simulink model "Exercitii_Laborator"  (R2016a)
settings: Solver=VariableStepDiscrete  StartTime=0.0  StopTime=40  RelTol=1e-3
undefined symbols (not defined in the file): m, n
settings Model: Creator=Cristina  LastModifiedBy=Cristina

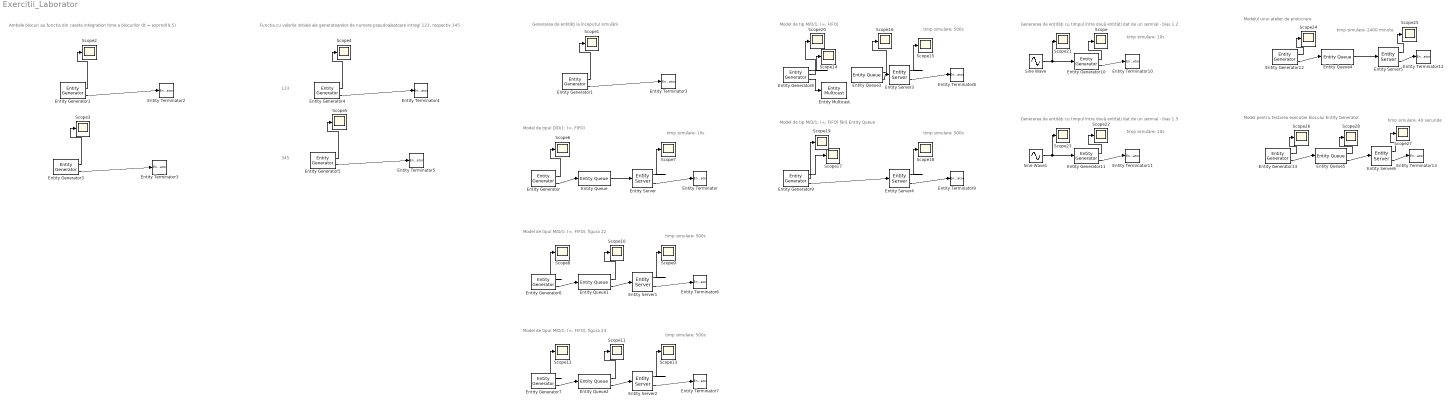
== system Exercitii_Laborator ==
  note: Model pentru testarea execuției blocului Entity Generator
  note: Generarea de entități cu timpul între două entități dat de un semnal - bias 1.2
  note: timp simulare: 10s
  note: Model de tipul D/D/1: (∞, FIFO)
  note: Generarea de entități la începutul simulării
  note: 345
  note: 123
  note: Functia cu valorile initiale ale generatoarelor de numere pseudoaleatoare intregi 123, respectiv
      | 345
  note: Ambele blocuri au functia din caseta integration time a blocurilor dt = exprnd(0.5)
  note: Model de tipul M/D/1: (∞, FIFO), figura 22
  note: timp simulare: 500s
  note: Model de tipul M/D/1: (∞, FIFO), figura 23
  note: timp simulare: 500s
  note: timp simulare: 500s
  note: Model de tip M/D/1; (∞, FIFO)
  note: timp simulare: 500s
  note: Model de tip M/D/1; (∞, FIFO) fără Entity Queue
  note: timp simulare: 10s
  note: Generarea de entități cu timpul între două entități dat de un semnal - bias 1.5
  note: timp simulare: 10s
  note: Modelul unui atelier de prelucrare
  note: timp simulare: 2400 minute
  note: timp simulare: 40 secunde
  Entity Generator : EntityGenerator  OutputPortMessageModes=n,m  NumberEntitiesDeparted=on  EntityType=Structured  EntityTypeName=Entity
      settings: OutputPortMap=o0,o3
  Entity Generator1 : EntityGenerator  OutputPortMessageModes=n,m  TimeSource=MATLAB action  IntergenerationTimeAction=|  NumberEntitiesDeparted=on  EntityType=Structured  EntityTypeName=Entity
      | persistent count
      | if (isempty(count))
      |     count = 1;
      | end
      | 
      | if count < 10
      |     dt = 0;
      |     count = count + 1;
      | else
      |     dt = inf;
      | end
      settings: OutputPortMap=o0,o3
  Entity Generator10 : EntityGenerator  OutputPortMessageModes=n,m  TimeSource=Signal port  NumberEntitiesDeparted=on  EntityType=Structured  EntityTypeName=Entity
      settings: InputPortMap=u1  OutputPortMap=o0,o3
  Entity Generator11 : EntityGenerator  OutputPortMessageModes=n,m  TimeSource=Signal port  NumberEntitiesDeparted=on  EntityType=Structured  EntityTypeName=Entity
      settings: InputPortMap=u1  OutputPortMap=o0,o3
  Entity Generator12 : EntityGenerator  OutputPortMessageModes=n,m  TimeSource=MATLAB action  IntergenerationTimeAction=|  AverageIntergenerationTime=on  EntityType=Structured  EntityTypeName=Entity
      | persistent init
      | if (isempty(init))
      |     rng(1957);
      |     init = true;
      | end
      | dt = 1 + rand * 12;
      settings: OutputPortMap=o2,o3
  Entity Generator13 : EntityGenerator  OutputPortMessageModes=n,m  IntergenerationTimeAction=|  NumberEntitiesDeparted=on  EntityType=Structured  EntityTypeName=Entity
      | persistent init
      | if (isempty(init))
      |     rng(1957);
      |     init = true;
      | end
      | dt = 1 + rand * 12;
      settings: OutputPortMap=o0,o3
  Entity Generator2 : EntityGenerator  OutputPortMessageModes=n,m  TimeSource=MATLAB action  IntergenerationTimeAction=dt = exprnd(0.5);  NumberEntitiesDeparted=on  EntityType=Structured  EntityTypeName=Entity
      settings: OutputPortMap=o0,o3
  Entity Generator3 : EntityGenerator  OutputPortMessageModes=n,m  TimeSource=MATLAB action  IntergenerationTimeAction=dt = exprnd(0.5);  NumberEntitiesDeparted=on  EntityType=Structured  EntityTypeName=Entity
      settings: OutputPortMap=o0,o3
  Entity Generator4 : EntityGenerator  OutputPortMessageModes=n,m  TimeSource=MATLAB action  IntergenerationTimeAction=|  NumberEntitiesDeparted=on  EntityType=Structured  EntityTypeName=Entity
      | persistent init
      | if isempty(init)
      |     rng(123);
      |     init = true;
      | end
      | 
      | dt = exprnd(0.5);
      settings: OutputPortMap=o0,o3
  Entity Generator5 : EntityGenerator  OutputPortMessageModes=n,m  TimeSource=MATLAB action  IntergenerationTimeAction=|  NumberEntitiesDeparted=on  EntityType=Structured  EntityTypeName=Entity
      | persistent init
      | if isempty(init)
      |     rng(345);
      |     init = true;
      | end
      | 
      | dt = exprnd(0.5);
      settings: OutputPortMap=o0,o3
  Entity Generator6 : EntityGenerator  OutputPortMessageModes=n,m  TimeSource=MATLAB action  IntergenerationTimeAction=dt = exprnd(0.5);  AverageIntergenerationTime=on  EntityType=Structured  EntityTypeName=Entity
      settings: OutputPortMap=o2,o3
  Entity Generator7 : EntityGenerator  OutputPortMessageModes=n,m  TimeSource=MATLAB action  IntergenerationTimeAction=|  AverageIntergenerationTime=on  EntityType=Structured  EntityTypeName=Entity
      | persistent init
      | if (isempty(init))
      |     rng(1437);
      |     init = true;
      | end
      | dt = exprnd(0.5);
      settings: OutputPortMap=o2,o3
  Entity Generator8 : EntityGenerator  OutputPortMessageModes=n,n,m  TimeSource=MATLAB action  IntergenerationTimeAction=|  NumberEntitiesDeparted=on  AverageIntergenerationTime=on  EntityType=Structured  EntityTypeName=Entity
      | persistent init
      | if (isempty(init))
      |     rng(1437);
      |     init = true;
      | end
      | dt = exprnd(0.5);
      settings: OutputPortMap=o0,o2,o3
  Entity Generator9 : EntityGenerator  OutputPortMessageModes=n,n,m  TimeSource=MATLAB action  IntergenerationTimeAction=|  NumberEntitiesDeparted=on  AverageIntergenerationTime=on  EntityType=Structured  EntityTypeName=Entity
      | persistent init
      | if (isempty(init))
      |     rng(1437);
      |     init = true;
      | end
      | dt = exprnd(0.5);
      settings: OutputPortMap=o0,o2,o3
  Entity Multicast : EntityMulticast  InputPortMessageModes=m
  Entity Queue : EntityQueue  InputPortMessageModes=m  OutputPortMessageModes=m
      settings: OutputPortMap=o5
  Entity Queue1 : EntityQueue  InputPortMessageModes=m  OutputPortMessageModes=n,m  NumberEntitiesInBlock=on
      settings: OutputPortMap=o1,o5
  Entity Queue2 : EntityQueue  InputPortMessageModes=m  OutputPortMessageModes=n,m  NumberEntitiesInBlock=on
      settings: OutputPortMap=o1,o5
  Entity Queue3 : EntityQueue  OutputPortMessageModes=n,m  EntityArrivalSource=Multicast  NumberEntitiesInBlock=on
      settings: OutputPortMap=o1,o5
  Entity Queue4 : EntityQueue  InputPortMessageModes=m  OutputPortMessageModes=m
      settings: OutputPortMap=o5
  Entity Queue5 : EntityQueue  InputPortMessageModes=m  OutputPortMessageModes=n,m  Capacity=10  NumberEntitiesInBlock=on
      settings: OutputPortMap=o1,o5
  Entity Server : EntityServer  InputPortMessageModes=m  OutputPortMessageModes=n,m  Capacity=1  NumberEntitiesDeparted=on
      settings: OutputPortMap=o0,o9
  Entity Server{1..4} (4 alike) : EntityServer  InputPortMessageModes=m  OutputPortMessageModes=n,m  Capacity=1  ServiceTimeValue=0.5  AverageWait=on
      settings: OutputPortMap=o4,o9
  Entity Server5 : EntityServer  InputPortMessageModes=m  OutputPortMessageModes=n,m  Capacity=1  ServiceTimeSource=MATLAB action  ServiceTimeAction=|  AverageWait=on
      | persistent init
      | if (isempty(init))
      |     rng(2347);
      |     init = true;
      | end
      | dt = 3.5 + rand * 3;
      settings: OutputPortMap=o4,o9
  Entity Server6 : EntityServer  InputPortMessageModes=m  OutputPortMessageModes=n,m  Capacity=1  ServiceTimeValue=2  ServiceTimeAction=|  NumberEntitiesDeparted=on
      | persistent init
      | if (isempty(init))
      |     rng(2347);
      |     init = true;
      | end
      | dt = 3.5 + rand * 3;
      settings: OutputPortMap=o0,o9
  Entity Terminator{,1..13} (14 alike) : EntityTerminator  InputPortMessageModes=m
  Scope{,1..28} (29 alike) : Scope
  Sine Wave : Sin  Bias=1.2  Frequency=1.2  SampleTime=0
  Sine Wave1 : Sin  Bias=1.5  Frequency=1.2  SampleTime=0
  wires:
  Entity Generator2/2 -> Entity Terminator2/1
  Entity Generator2/1 -> Scope2/1
  Entity Generator3/2 -> Entity Terminator3/1
  Entity Generator3/1 -> Scope3/1
  Entity Generator4/2 -> Entity Terminator4/1
  Entity Generator4/1 -> Scope4/1
  Entity Generator5/2 -> Entity Terminator5/1
  Entity Generator5/1 -> Scope5/1
  Entity Generator1/2 -> Entity Terminator1/1
  Entity Generator1/1 -> Scope1/1
  Entity Generator/2 -> Entity Queue/1
  Entity Queue/1 -> Entity Server/1
  Entity Server/2 -> Entity Terminator/1
  Entity Generator/1 -> Scope6/1
  Entity Server/1 -> Scope7/1
  Entity Generator6/2 -> Entity Queue1/1
  Entity Queue1/2 -> Entity Server1/1
  Entity Server1/2 -> Entity Terminator6/1
  Entity Generator6/1 -> Scope8/1
  Entity Server1/1 -> Scope9/1
  Entity Queue1/1 -> Scope10/1
  Entity Generator7/2 -> Entity Queue2/1
  Entity Queue2/2 -> Entity Server2/1
  Entity Server2/2 -> Entity Terminator7/1
  Entity Generator7/1 -> Scope12/1
  Entity Server2/1 -> Scope13/1
  Entity Queue2/1 -> Scope11/1
  Entity Queue3/2 -> Entity Server3/1
  Entity Server3/2 -> Entity Terminator8/1
  Entity Generator8/1 -> Scope14/1
  Entity Server3/1 -> Scope15/1
  Entity Generator8/3 -> Entity Multicast/1
  Entity Queue3/1 -> Scope16/1
  Entity Server4/2 -> Entity Terminator9/1
  Entity Generator9/1 -> Scope17/1
  Entity Server4/1 -> Scope18/1
  Entity Generator9/3 -> Entity Server4/1
  Entity Generator9/2 -> Scope19/1
  Entity Generator8/2 -> Scope20/1
  Sine Wave/1 -> Scope21/1, Entity Generator10/1
  Entity Generator10/2 -> Entity Terminator10/1
  Entity Generator10/1 -> Scope/1
  Sine Wave1/1 -> Entity Generator11/1, Scope23/1
  Entity Generator11/2 -> Entity Terminator11/1
  Entity Generator11/1 -> Scope22/1
  Entity Generator12/2 -> Entity Queue4/1
  Entity Queue4/1 -> Entity Server5/1
  Entity Server5/2 -> Entity Terminator12/1
  Entity Generator12/1 -> Scope24/1
  Entity Server5/1 -> Scope25/1
  Entity Generator13/2 -> Entity Queue5/1
  Entity Queue5/2 -> Entity Server6/1
  Entity Server6/2 -> Entity Terminator13/1
  Entity Generator13/1 -> Scope26/1
  Entity Server6/1 -> Scope27/1
  Entity Queue5/1 -> Scope28/1
